simulink model "AreaCoverageTestHarness"  (R2016a)
settings: Solver=FixedStepDiscrete  StartTime=0.0  StopTime=16  FixedStep=0.005  RelTol=1e-3
undefined symbols (not defined in the file): EAST, ERRVAL, INIT_COMP_VALUE, INIT_X, INIT_Y, MAX_SPEED, NORTH, PLOT_SAMPLE, ROB_LENG, ROB_WHEEL_R, room, roomSize, SAMPLE_TIME, sigbuilder_block, SOUTH, STEP_SIZE, WEST
(part 2 of 2)

== stateflow chart AreaCoverageTestHarness/Robot/ULS_Calc/Chart ==
  state WestCalc
    entry:
    leftCounter = y-1;
    rightCounter = y-1;
    ULSL = 0;
    ULSR = 0;
    startLeft = true;
    startRight = true;
    state ULSL [parallel]
      settings: executionOrder=2
      (history)
      state ULSL_Calc
      state Hit
      WestCalc.ULSL.ULSL_Calc -> (junction 148) : [leftCounter+1 <= roomSize]{leftCounter++;}
      (default) -> WestCalc.ULSL.ULSL_Calc
      (junction 148) -> WestCalc.ULSL.Hit [order 1] : [room[leftCounter][x-1] == 0]
      (junction 148) -> WestCalc.ULSL.ULSL_Calc [order 2] : [room[leftCounter][x-1] == 255]
          | /ULSL++;
      WestCalc.ULSL.Hit -> WestCalc.ULSL.ULSL_Calc : [startLeft]/startLeft = false;
    state ULSR [parallel]
      settings: executionOrder=1
      (history)
      state ULSR_Calc1
      state Hit
      WestCalc.ULSR.ULSR_Calc1 -> (junction 147) : [rightCounter - 1 >= 0]{rightCounter--;}
      (default) -> WestCalc.ULSR.ULSR_Calc1
      (junction 147) -> WestCalc.ULSR.Hit [order 1] : [room[rightCounter][x-1] == 0]
      (junction 147) -> WestCalc.ULSR.ULSR_Calc1 [order 2] : [room[rightCounter][x-1] == 255]
          | /ULSR++;
      WestCalc.ULSR.Hit -> WestCalc.ULSR.ULSR_Calc1 : [startRight]/startRight = false;
  state NorthCalc
    entry:
    leftCounter = x-1;
    rightCounter = x-1;
    ULSL = 0;
    ULSR = 0;
    startLeft = true;
    startRight = true;
    state ULSL [parallel]
      settings: executionOrder=2
      (history)
      state ULSL_Calc
      state Hit
      NorthCalc.ULSL.ULSL_Calc -> (junction 193) : [leftCounter - 1 >= 0]{leftCounter--;}
      (default) -> NorthCalc.ULSL.ULSL_Calc
      (junction 193) -> NorthCalc.ULSL.Hit [order 1] : [room[y-1][leftCounter] == 0]
      (junction 193) -> NorthCalc.ULSL.ULSL_Calc [order 2] : [room[y-1][leftCounter] == 255]
          | /ULSL++;
      NorthCalc.ULSL.Hit -> NorthCalc.ULSL.ULSL_Calc : [startLeft]/startLeft = false;
    state ULSR [parallel]
      settings: executionOrder=1
      (history)
      state ULSR_Calc
      state Hit
      NorthCalc.ULSR.ULSR_Calc -> (junction 206) : [rightCounter + 1 <= roomSize]{rightCounter++;}
      (default) -> NorthCalc.ULSR.ULSR_Calc
      (junction 206) -> NorthCalc.ULSR.Hit [order 1] : [room[y - 1][rightCounter] == 0]
      (junction 206) -> NorthCalc.ULSR.ULSR_Calc [order 2] : [room[y - 1][rightCounter] == 255]
          | /ULSR++;
      NorthCalc.ULSR.Hit -> NorthCalc.ULSR.ULSR_Calc : [startRight]/startRight = false;
  state CalcHeading
    (default) -> (junction 2)
    (junction 2) -> (junction 3) [order 1] : [(theta <= 270+ERRVAL) && (theta >= 270 - ERRVAL)]//NORTH
    (junction 2) -> (junction 4) [order 2]
    (junction 3) -> (junction 17) : {heading = NORTH;}
    (junction 4) -> (junction 5) [order 1] : [(theta <= 90+ERRVAL) && (theta >= 90-ERRVAL)]//SOUTH
    (junction 4) -> (junction 6) [order 2]
    (junction 5) -> (junction 16) : {heading = SOUTH;}
    (junction 6) -> (junction 7) [order 1] : [(theta <= 0+ERRVAL) || (theta >= 360-ERRVAL)]//EAST
    (junction 6) -> (junction 8) [order 2]
    (junction 7) -> (junction 15) : {heading = EAST;}
    (junction 8) -> (junction 9) [order 1] : [(theta <= 180+ERRVAL) && (theta >= 180-ERRVAL)]//WEST
    (junction 8) -> (junction 10) [order 2] : {heading = NONE;}
    (junction 9) -> (junction 14) : {heading = WEST;}
    (junction 10) -> (junction 11) [order 2] : [Vr == Vl]
    (junction 11) -> (junction 13) : {wrongHeading_BOOL = true;}
    (junction 10) -> (junction 12) [order 1]
    (junction 13) -> (junction 12)
    (junction 14) -> (junction 13) : {wrongHeading_BOOL = false;}
    (junction 15) -> (junction 14)
    (junction 16) -> (junction 15)
    (junction 17) -> (junction 16)
    (junction 12) -> (junction 18)
  state EastCalc
    entry:
    leftCounter = y-1;
    rightCounter = y-1;
    ULSL = 0;
    ULSR = 0;
    startLeft = true;
    startRight = true;
    state ULSL [parallel]
      settings: executionOrder=2
      (history)
      state ULSL_Calc
      state Hit
      EastCalc.ULSL.ULSL_Calc -> (junction 172) : [leftCounter - 1 >= 0]{leftCounter--;}
      (default) -> EastCalc.ULSL.ULSL_Calc
      (junction 172) -> EastCalc.ULSL.Hit [order 1] : [room[leftCounter][x-1] == 0]
      (junction 172) -> EastCalc.ULSL.ULSL_Calc [order 2] : [room[leftCounter][x-1] == 255]
          | /ULSL++;
      EastCalc.ULSL.Hit -> EastCalc.ULSL.ULSL_Calc : [startLeft]/startLeft = false;
    state ULSR [parallel]
      settings: executionOrder=1
      (history)
      state ULSR_Calc1
      state Hit
      EastCalc.ULSR.ULSR_Calc1 -> (junction 185) : [rightCounter + 1 <= roomSize]{rightCounter++;}
      (default) -> EastCalc.ULSR.ULSR_Calc1
      (junction 185) -> EastCalc.ULSR.Hit [order 1] : [room[rightCounter][x-1] == 0]
      (junction 185) -> EastCalc.ULSR.ULSR_Calc1 [order 2] : [room[rightCounter][x-1] == 255]
          | /ULSR++;
      EastCalc.ULSR.Hit -> EastCalc.ULSR.ULSR_Calc1 : [startRight]/startRight = false;
  state SouthCalc
    entry:
    leftCounter = x-1;
    rightCounter = x-1;
    ULSL = 0;
    ULSR = 0;
    startLeft = true;
    startRight = true;
    state ULSL [parallel]
      settings: executionOrder=2
      (history)
      state ULSL_Calc
      state Hit
      SouthCalc.ULSL.ULSL_Calc -> (junction 226) : [leftCounter + 1 <= roomSize]{leftCounter++;}
      (default) -> SouthCalc.ULSL.ULSL_Calc
      (junction 226) -> SouthCalc.ULSL.Hit [order 1] : [room[y-1][leftCounter] == 0]
      (junction 226) -> SouthCalc.ULSL.ULSL_Calc [order 2] : [room[y-1][leftCounter] == 255]
          | /ULSL++;
      SouthCalc.ULSL.Hit -> SouthCalc.ULSL.ULSL_Calc : [startLeft]/startLeft = false;
    state ULSR [parallel]
      settings: executionOrder=1
      (history)
      state ULSR_Calc
      state Hit
      SouthCalc.ULSR.ULSR_Calc -> (junction 213) : [rightCounter - 1 >= 0]{rightCounter--;}
      (default) -> SouthCalc.ULSR.ULSR_Calc
      (junction 213) -> SouthCalc.ULSR.Hit [order 1] : [room[y - 1][rightCounter] == 0]
      (junction 213) -> SouthCalc.ULSR.ULSR_Calc [order 2] : [room[y - 1][rightCounter] == 255]
          | /ULSR++;
      SouthCalc.ULSR.Hit -> SouthCalc.ULSR.ULSR_Calc : [startRight]/startRight = false;
  (default) -> CalcHeading
  CalcHeading -> WestCalc [order 1] : [heading == WEST]/readingReady = false;
  CalcHeading -> NorthCalc [order 4] : [heading == NORTH]/readingReady = false;
  WestCalc -> (junction 154)
  (junction 154) -> CalcHeading : [(room[rightCounter][x-1] == 0)...
      |  &&(room[leftCounter][x-1] == 0)
      | ]/readingReady = true;
  NorthCalc -> (junction 117)
  EastCalc -> (junction 154)
  (junction 117) -> CalcHeading : [(room[y-1][rightCounter] == 0)...
      |  &&(room[y-1][leftCounter] == 0)]
      | /readingReady = true;
  SouthCalc -> (junction 117)
  CalcHeading -> EastCalc [order 2] : [heading == EAST]/readingReady = false;
  CalcHeading -> SouthCalc [order 3] : [heading == SOUTH]/readingReady = false;
  data: ERRVAL input; NORTH input; SOUTH input; EAST input; WEST input; NONE input; room input size=[roomSize roomSize]; heading local int16; theta input; Vl input; Vr input; roomSize input; x input; y input; wrongHeading_BOOL output double; ULSL output double; ULSR output double; leftCounter local double; rightCounter local double; startLeft local boolean; startRight local boolean; readingReady output boolean

== matlab function AreaCoverageTestHarness/Robot/MATLAB Function ==
  data: X input; Y input; Theta input; roomSize input; Event input
function PlotterFunc(X, Y, Theta, roomSize, Event)

lineLength = round(roomSize*0.12);
plotCounter = 0;
opleft = sind(Theta+90) * (lineLength/2);
    adjleft = cosd(Theta+90) * (lineLength/2);
    yend = Y + opleft;
    xend = X + adjleft;
    start = [X xend];
    finish = [Y yend];

    opright = sind(Theta-90) * (lineLength/2);
    adjright = cosd(Theta-90) * (lineLength/2);
    if Event
        plot(X, Y, '*', 'MarkerSize', 10);
        hold on
        plot(start, finish, 'LineWidth', 3)
        plot(xend, yend, 'or')
        yend = Y + opright;
        xend = X + adjright;
        start = [X xend];
        finish = [Y yend];
        plot(start, finish, 'LineWidth', 3)
        plot(xend, yend, 'or')
        hold off
        xlim([0 roomSize]);
        ylim([0 roomSize]);
        grid on
        grid minor
        plotCounter = 0;
    end
    plotCounter = plotCounter + 1;
    pause(0.001);

== stateflow chart AreaCoverageTestHarness/Robot/PlotSampler ==
  (default) -> (junction 1)
  (junction 1) -> (junction 3) : {counter = counter + 1;...
      | Event_BOOL = false;}
  (junction 3) -> (junction 5) [order 1] : [counter >= PLOT_SAMPLE]
  (junction 3) -> (junction 9) [order 2] : /{Event_BOOL = false;}
  (junction 5) -> (junction 7) : {counter = 0;...
      | Event_BOOL = true;}
  (junction 7) -> (junction 9)
  data: counter local uint8; Event_BOOL output boolean; PLOT_SAMPLE input

== stateflow chart AreaCoverageTestHarness/Robot/EncoderTicksGenerator/SquareWaveCreatorLeft ==
  state BulbOn
    state Off
      entry:
      counter = 0;
      encoderTicks_BOOL = false;
      du:
      counter++;
    state On
      entry:
      counter = 0;
      encoderTicks_BOOL = true;
      du:
      counter++;
    (default) -> Off
    On -> Off : [counter >= 100]/counter = 0;
    Off -> On : [counter >= 100]/counter = 0;
  state BulbOff
    entry:
    encoderTicks_BOOL = 0;
  (default) -> BulbOff
  BulbOff -> BulbOn : [ControlSignal_BOOL_in]
  BulbOn -> BulbOff : [!ControlSignal_BOOL_in]
  data: ControlSignal_BOOL_in input; encoderTicks_BOOL output boolean; counter local uint16
